simulink model "afferent_step_response"  (Simulink 6.6)
settings: Solver=ode45  StartTime=0.0  StopTime=10.0  RelTol=1e-3
values from neighbouring files (symbols this model uses):
  T = 0.015    [canal_afferent_step_response.m]
  T1 = 5.7    [canal_afferent_step_response.m]
  T2 = 0.003    [canal_afferent_step_response.m]
  Ts = simoutTP    [canal_afferent_step_response.m]
settings Model: Creator=adams  LastModifiedBy=adams  ExtModeAutoUpdateStatusClock=off
settings DebuggingCC: SignalResolutionControl=TryResolveAllWithWarning  MultiTaskDSMMsg=warning  MultiTaskCondExecSysMsg=none  StrictBusMsg=None
settings RTWCC: IncludeERTFirstTime=on

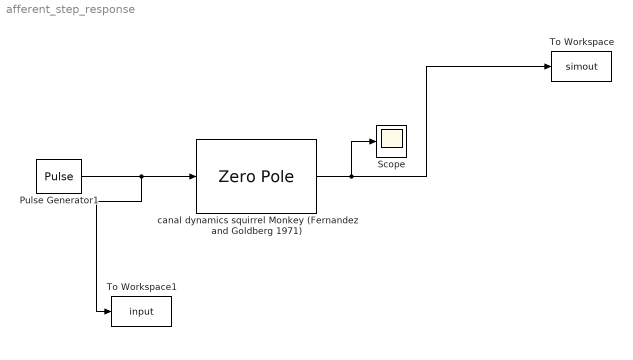
== system afferent_step_response ==
  Pulse Generator1 : DiscretePulseGenerator  PulseType=Time based  Period=100  PulseWidth=50  PhaseDelay=10
  Scope : Scope
  To Workspace : ToWorkspace  VariableName=simout  SampleTime=Ts  SaveFormat=Array
  To Workspace1 : ToWorkspace  VariableName=input  SampleTime=Ts  SaveFormat=Array
  canal dynamics squirrel Monkey (Fernandez and Goldberg 1971) : ZeroPole  Zeros=[0 -1/T]  Poles=[-1/T1 -1/T2]  Gain=[T/(T1*T2)]
  wires:
  Pulse Generator1/1 -> To Workspace1/1, canal dynamics squirrel Monkey (Fernandez and Goldberg 1971)/1
  canal dynamics squirrel Monkey (Fernandez and Goldberg 1971)/1 -> To Workspace/1, Scope/1
